simulink model "trike_states_2018b"  (R2019b)
settings: Solver=VariableStepAuto  StartTime=0.0  StopTime=10.0  RelTol=1e-3
settings Model: Creator=uidr9910  LastModifiedBy=uidr9910

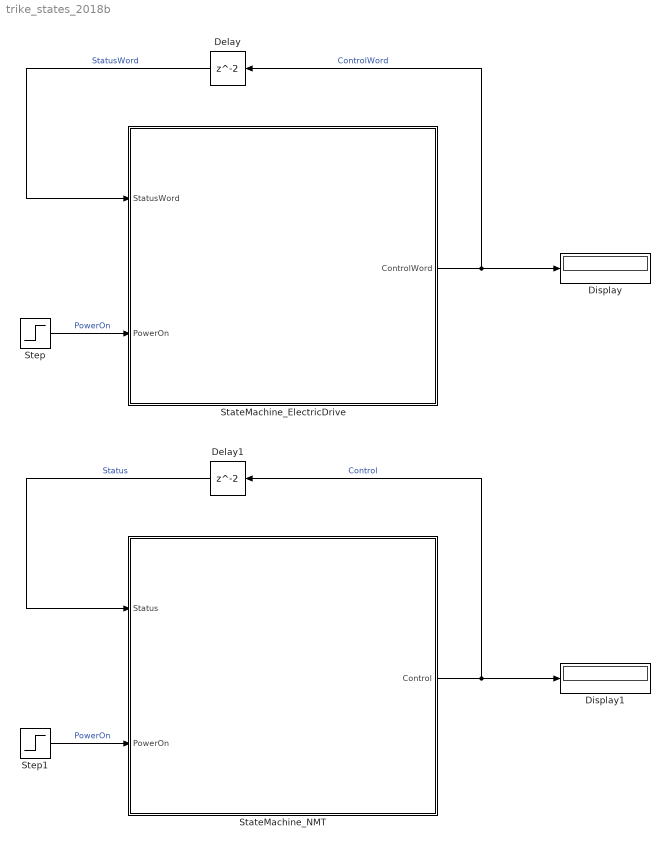
== system trike_states_2018b ==
  Delay : Delay  InitialCondition=0
  Delay1 : Delay  InitialCondition=0
  Display : Display
  Display1 : Display
  StateMachine_ElectricDrive : Stateflow chart  TreatAsAtomicUnit=on
  StateMachine_NMT : Stateflow chart  TreatAsAtomicUnit=on
  Step : Step  Time=5  Before=1  After=0  SampleTime=0
  Step1 : Step  Time=5  Before=1  After=0  SampleTime=0
  wires:
  StateMachine_ElectricDrive/1(ControlWord) -> Delay/1, Display/1  "ControlWord"
  Delay/1 -> StateMachine_ElectricDrive/1(StatusWord)  "StatusWord"
  Step/1 -> StateMachine_ElectricDrive/2(PowerOn)  "PowerOn"
  Step1/1 -> StateMachine_NMT/2(PowerOn)  "PowerOn"
  Delay1/1 -> StateMachine_NMT/1(Status)  "Status"
  StateMachine_NMT/1(Control) -> Display1/1, Delay1/1  "Control"

== stateflow chart trike_states_2018b/StateMachine_NMT ==
  state Init
    entry:
    x00=0;
    x01=3;
    x1=6;
    x2=15;
    x3=3;
  state ResetApplication
    entry:
    Control=x00;
  state ResetCommunication
    entry:
    Control=x01;
  state Pre_Operational
    entry:
    Control=x1;
  state Operational
    entry:
    Control=x2;
  state Stopped
    entry:
    Control=x3;
  (default) -> Init
  Stopped -> ResetApplication [order 1] : [Status==x5 && PowerOn==0]{after(10,tick)}
  Init -> ResetApplication
  Operational -> ResetApplication [order 3] : [Status==x4 && PowerOn==0]{after(10,tick)}
  Pre_Operational -> ResetApplication [order 3] : [Status==x3 && PowerOn==0]{after(10,tick)}
  Pre_Operational -> Stopped [order 4] : [Status==x4 && PowerOn==0]{after(10,tick)}
  ResetApplication -> ResetCommunication : [Status==x1 && PowerOn==1]{after(10,tick)}
  Operational -> Pre_Operational [order 1] : [Status==x4 && PowerOn==0]{after(10,tick)}
  ResetCommunication -> Pre_Operational : [Status==x2 && PowerOn==1]{after(10,tick)}
  Stopped -> Operational [order 3] : [Status==x4 && PowerOn==0]{after(10,tick)}
  Pre_Operational -> Operational [order 2] : [Status==x3 && PowerOn==1]{after(10,tick)}
  Operational -> Stopped [order 2] : [Status==x4 && PowerOn==0]{after(10,tick)}
  Pre_Operational -> ResetCommunication [order 1] : [Status==x3 && PowerOn==0]{after(10,tick)}
  Operational -> ResetCommunication [order 4] : [Status==x4 && PowerOn==0]{after(10,tick)}
  Stopped -> ResetCommunication [order 2] : [Status==x4 && PowerOn==0]{after(10,tick)}
  Stopped -> Pre_Operational [order 4] : [Status==x4 && PowerOn==0]{after(10,tick)}
  data: Control output; Status input; x1 local; x2 local; x3 local; x00 local; x01 local; PowerOn input

== stateflow chart trike_states_2018b/StateMachine_ElectricDrive ==
  state Init
    entry:
    x1=0;
    x2=3;
    x3=6;
    x4=15;
    x5=3;
  state SwitchOn_Disabled
    entry:
    ControlWord=x1;
  state Ready_to_SwitchOn
    entry:
    ControlWord=x2;
  state SwitchOn
    entry:
    ControlWord=x3;
  state OperationEnable
    entry:
    ControlWord=x4;
  state QuickStop
    entry:
    ControlWord=x5;
  (default) -> Init
  Init -> SwitchOn_Disabled
  SwitchOn_Disabled -> Ready_to_SwitchOn : [StatusWord==x1 && PowerOn==1]{after(10,tick)}
  Ready_to_SwitchOn -> SwitchOn_Disabled [order 1] : [StatusWord==x2 && PowerOn==0]{after(10,tick)}
  SwitchOn -> Ready_to_SwitchOn [order 1] : [StatusWord==x3 && PowerOn==0]{after(10,tick)}
  Ready_to_SwitchOn -> SwitchOn [order 2] : [StatusWord==x2 && PowerOn==1]{after(10,tick)}
  SwitchOn -> SwitchOn_Disabled [order 3] : [StatusWord==x3 && PowerOn==0]{after(10,tick)}
  OperationEnable -> SwitchOn [order 1] : [StatusWord==x4 && PowerOn==0]{after(10,tick)}
  SwitchOn -> OperationEnable [order 2] : [StatusWord==x3 && PowerOn==1]{after(10,tick)}
  OperationEnable -> SwitchOn_Disabled [order 3] : [StatusWord==x4 && PowerOn==0]{after(10,tick)}
  OperationEnable -> QuickStop [order 2] : [StatusWord==x4 && PowerOn==0]{after(10,tick)}
  QuickStop -> SwitchOn_Disabled : [StatusWord==x5 && PowerOn==0]{after(10,tick)}
  data: ControlWord output; StatusWord input; x1 local; x2 local; x3 local; x4 local; x5 local; PowerOn input
